simulink model "SF109A_ElecPwrCns"  (R2013b)
settings: Solver=FixedStepDiscrete  SolverMode=SingleTasking  StartTime=0.0  StopTime=1  FixedStep=0.002  RelTol=1e-3
values from neighbouring files (symbols this model uses):
  ARCHGLBPRM_HALFSQRT3_ULS_F32 = DataDict.Constant    [SF109A_ElecPwrCns_DataDict.m]
  ELECINPPWRESTIMHILIM_WATT_F32 = DataDict.Constant    [SF109A_ElecPwrCns_DataDict.m]
  ELECINPPWRESTIMLOLIM_WATT_F32 = DataDict.Constant    [SF109A_ElecPwrCns_DataDict.m]
  ElecPwrCnsCtrlrInpR = DataDict.Calibration    [SF109A_ElecPwrCns_DataDict.m]
  ElecPwrCnsPrstcPwrLoss = DataDict.Calibration    [SF109A_ElecPwrCns_DataDict.m]
  SPLYCURRESTIMHILIM_AMPR_F32 = DataDict.Constant    [SF109A_ElecPwrCns_DataDict.m]
  SPLYCURRESTIMLOLIM_AMPR_F32 = DataDict.Constant    [SF109A_ElecPwrCns_DataDict.m]
libraries: simulink x1
settings Model: LastModifiedBy=DZ1YRM
settings SolverCC: AutoInsertRateTranBlk=on  InsertRTBMode=Always
settings DataIOCC: LimitDataPoints=off  SaveFormat=Structure  ReturnWorkspaceOutputs=on
settings OptimizationCC: BlockReduction=off  InlineParams=on  ZeroExternalMemoryAtStartup=off  ZeroInternalMemoryAtStartup=off  OptimizeModelRefInitCode=on  LifeSpan=1
settings DebuggingCC: SignalInfNanChecking=error  SignalRangeChecking=warning  UnderspecifiedInitializationDetection=Simplified  SolverPrmCheckMsg=error  InheritedTsInSrcMsg=error  DiscreteInheritContinuousMsg=error  SingleTaskRateTransMsg=error  TasksWithSamePriorityMsg=error  SigSpecEnsureSampleTimeMsg=error  CheckMatrixSingularityMsg=error  ParameterUnderflowMsg=error  ParameterPrecisionLossMsg=error  ParameterTunabilityLossMsg=error  FixptConstUnderflowMsg=warning  FixptConstOverflowMsg=warning  VectorMatrixConversionMsg=error  SignalLabelMismatchMsg=error  UnconnectedInputMsg=error  UnconnectedOutputMsg=error  UnconnectedLineMsg=error  SFcnCompatibilityMsg=error  UniqueDataStoreMsg=warning  BusObjectLabelMismatch=error  RootOutportRequireBusObject=error  AssertControl=DisableAll  ModelReferenceIOMsg=error  ModelReferenceVersionMismatchMessage=warning  ModelReferenceIOMismatchMessage=error  ModelReferenceCSMismatchMessage=warning  ModelReferenceDataLoggingMessage=error  StateNameClashWarn=warning  StrictBusMsg=ErrorOnBusTreatedAsVector  NonBusSignalsTreatedAsBus=error  SFUnexpectedBacktrackingDiag=error  SFInvalidInputDataAccessInChartInitDiag=error  SFNoUnconditionalDefaultTransitionDiag=error  SFTransitionOutsideNaturalParentDiag=error  SFUnconditionalTransitionShadowingDiag=error  SFUndirectedBroadcastEventsDiag=error
settings ModelReferenceCC: ModelReferenceNumInstancesAllowed=Single
settings RTWCC: SystemTargetFile=autosar.tlc  GenCodeOnly=on  TemplateMakefile=ert_default_tmf  Description=AUTOSAR  GenerateReport=on  ProcessScript=autosar_make_rtw_hook  LaunchReport=on
settings CodeAppCC: GenerateComments=off  IgnoreCustomStorageClasses=off  CustomSymbolStrType=$N$R$M  CustomSymbolStrBlkIO=$N$M  SimulinkBlockComments=off
settings STFCustomTargetCC: ParMdlRefBuildCompliant=on  CompOptLevelCompliant=on  IncludeMdlTerminateFcn=off  CombineOutputUpdateFcns=on  SuppressErrorStatus=on  ERTFirstTimeCompliant=on  ERTCustomFileBanners=on  SupportNonFinite=off  SupportComplex=off  SupportContinuousTime=off  SupportNonInlinedSFcns=off  MATLABClassNameForMDSCustomization=Simulink.SoftwareTarget.ERTCustomization  AutosarCompliant=on  GRTInterface=off  SystemTargetFile=autosar.tlc
settings ERTTargetCC: CodeReplacementLibrary=ANSI_C  ConcurrentExecutionCompliant=off  IncludeMdlTerminateFcn=off  SuppressErrorStatus=on  SupportNonFinite=off  SupportComplex=off  ModelStepFunctionPrototypeControlCompliant=off  CPPClassGenCompliant=off  AutosarCompliant=on  InlinedParameterPlacement=NonHierarchical  ERTCustomFileTemplate=example_file_process.tlc  EnableUserReplacementTypes=on

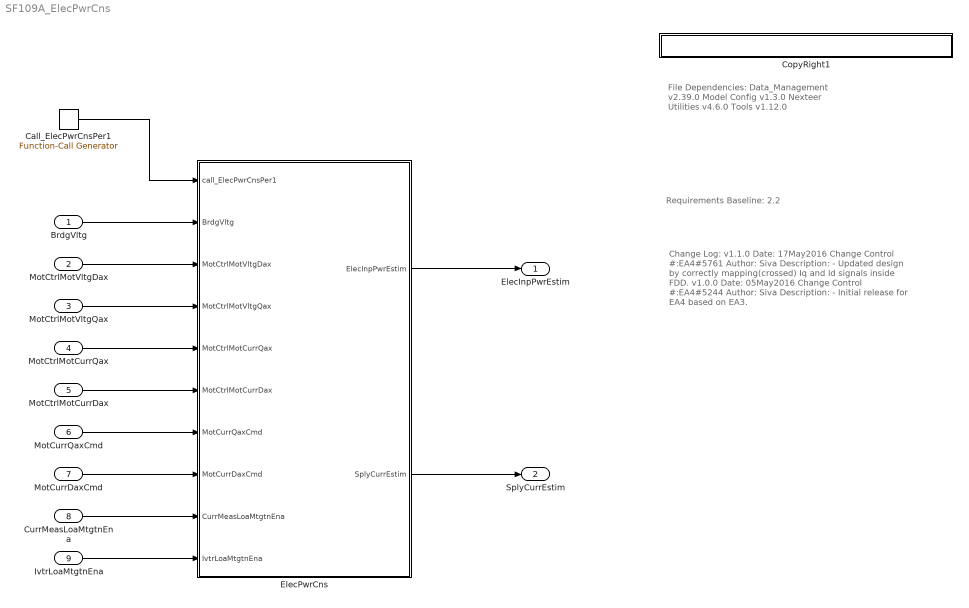
== system SF109A_ElecPwrCns ==
  note: File Dependencies:
      |
      | Data_Management v2.39.0
      | Model Config v1.3.0
      | Nexteer Utilities v4.6.0
      | Tools v1.12.0
  note: Requirements Baseline: 2.2
  note: Change Log:
      |
      | v1.1.0
      | Date: 17May2016
      | Change Control #:EA4#5761
      | Author: Siva
      | Description:
      | - Updated design by correctly mapping(crossed)
      |   Iq and Id signals inside FDD.
      |
      |
      | v1.0.0
      | Date: 05May2016
      | Change Control #:EA4#5244
      | Author: Siva
      | Description:
      | - Initial release for EA4 based on EA3.
  BrdgVltg : Inport
  MotCtrlMotVltgDax : Inport  Port=2
  MotCtrlMotVltgQax : Inport  Port=3
  MotCtrlMotCurrQax : Inport  Port=4
  MotCtrlMotCurrDax : Inport  Port=5
  MotCurrQaxCmd : Inport  Port=6
  MotCurrDaxCmd : Inport  Port=7
  CurrMeasLoaMtgtnEna : Inport  Port=8
  IvtrLoaMtgtnEna : Inport  Port=9
  Call_ElecPwrCnsPer1 : simulink/Ports & Subsystems/Function-Call Generator  sample_time=0.01  numberOfIterations=1
  CopyRight1 : Subsystem  Description=|  mask(Copyright Information){none=on}
      | Copyright info block.                                               
      |                                                                     
      | Place copyright information at the top of every subsystem in design.
      mask prompts: none "No parameters"
      mask help: Place copyright information at the top of every subsystem in design.
      mask Display:
      | NxtrConf = 'Nexteer Confidential';
      | 
      | sys = bdroot; %handle for the current model ("system")
      | first = get_param(sys,'Created');
      | if(isempty(first))
      |     first = datestr(now,'yyyy');
      | else
      |     first = first(end-3:end);  %year is last four digits
      | end
      | 
      | last = get_param(sys,'LastModifiedDate');
      | if isempty(last)
      |     last = datestr(now,'yyyy');
      | else
      |     last = last(end-3:end);
      | end
      | 
      | if strcmp(first,last)
      |     fprintf('%s -- Copyright %s Nexteer',NxtrConf,first)
      | else
      |     fprintf('%s -- %s%s- %s Nexteer',NxtrConf,char(169),first,last)
      | end
  ElecPwrCns : Subsystem
  ElecInpPwrEstim : Outport
  SplyCurrEstim : Outport  Port=2
  wires:
  ElecPwrCns/1(ElecInpPwrEstim) -> ElecInpPwrEstim/1
  ElecPwrCns/2(SplyCurrEstim) -> SplyCurrEstim/1
  Call_ElecPwrCnsPer1/1 -> ElecPwrCns/1(call_ElecPwrCnsPer1)
  MotCtrlMotVltgDax/1 -> ElecPwrCns/3(MotCtrlMotVltgDax)
  MotCtrlMotCurrDax/1 -> ElecPwrCns/6(MotCtrlMotCurrDax)
  CurrMeasLoaMtgtnEna/1 -> ElecPwrCns/9(CurrMeasLoaMtgtnEna)
  IvtrLoaMtgtnEna/1 -> ElecPwrCns/10(IvtrLoaMtgtnEna)
  MotCurrDaxCmd/1 -> ElecPwrCns/8(MotCurrDaxCmd)
  MotCtrlMotVltgQax/1 -> ElecPwrCns/4(MotCtrlMotVltgQax)
  MotCurrQaxCmd/1 -> ElecPwrCns/7(MotCurrQaxCmd)
  BrdgVltg/1 -> ElecPwrCns/2(BrdgVltg)
  MotCtrlMotCurrQax/1 -> ElecPwrCns/5(MotCtrlMotCurrQax)

== system SF109A_ElecPwrCns/CopyRight1 ==

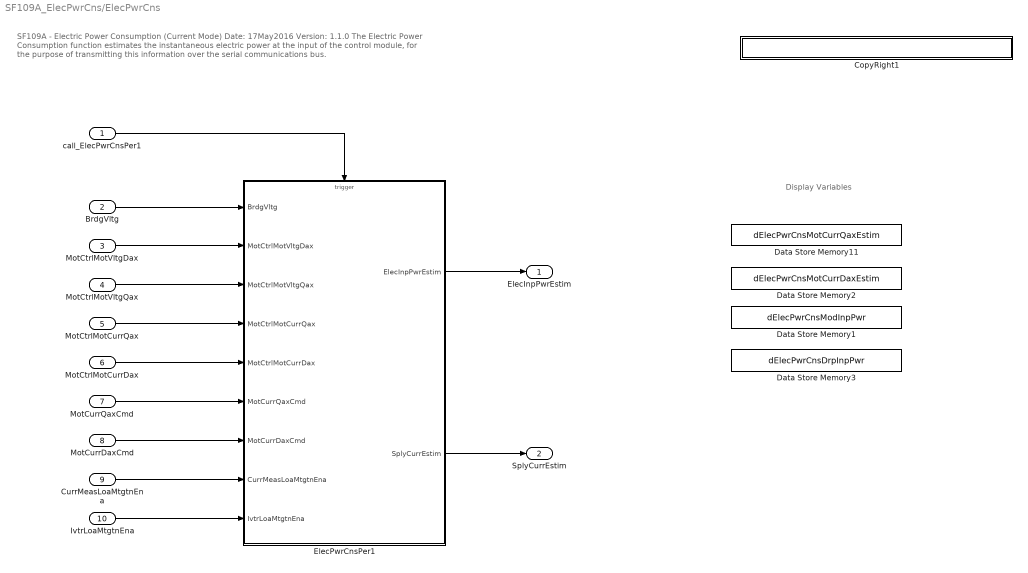
== system SF109A_ElecPwrCns/ElecPwrCns ==
  note: SF109A - Electric Power Consumption (Current Mode)
      | Date: 17May2016
      | Version: 1.1.0
      |
      | The Electric Power Consumption function estimates the instantaneous electric power at the input of the control module, for the purpose of transmitting this information
      | over the serial communications bus.
  note: Display Variables
  call_ElecPwrCnsPer1 : Inport  RequirementInfo={} %GIDa_da0c0603_8467_4dbe_980a_34e234362c51
  BrdgVltg : Inport  RequirementInfo="{'linktype_rmi_doors' '0000bb49 (/E-STEER Core/SubSystem Specifications/Application Functions/SF109A Electric Power Consumption )' '#SF109A_9' 'true' 'REQ:  SF109A_9' '' } %GIDa_cb384746_122a_4ac6_a5fd_4cc52726ee4f"  Port=2
  MotCtrlMotVltgDax : Inport  RequirementInfo="{'linktype_rmi_doors' '0000bb49 (/E-STEER Core/SubSystem Specifications/Application Functions/SF109A Electric Power Consumption )' '#SF109A_33' 'true' 'REQ:  SF109A_33' '' } %GIDa_0fee7270_14d1_452d_96a5_d6615c243f53"  Port=3
  MotCtrlMotVltgQax : Inport  RequirementInfo="{'linktype_rmi_doors' '0000bb49 (/E-STEER Core/SubSystem Specifications/Application Functions/SF109A Electric Power Consumption )' '#SF109A_32' 'true' 'REQ:  SF109A_32' '' } %GIDa_1366854d_cdb8_41c9_9ec7_b295409961f7"  Port=4
  MotCtrlMotCurrQax : Inport  RequirementInfo="{'linktype_rmi_doors' '0000bb49 (/E-STEER Core/SubSystem Specifications/Application Functions/SF109A Electric Power Consumption )' '#SF109A_34' 'true' 'REQ:  SF109A_34' '' } %GIDa_5e8aa2b9_a336_4638_be53_d49e57df33ab"  Port=5
  MotCtrlMotCurrDax : Inport  RequirementInfo="{'linktype_rmi_doors' '0000bb49 (/E-STEER Core/SubSystem Specifications/Application Functions/SF109A Electric Power Consumption )' '#SF109A_35' 'true' 'REQ:  SF109A_35' '' } %GIDa_7b415b12_f15f_4f64_9d4b_d3b77c1c51c9"  Port=6
  MotCurrQaxCmd : Inport  RequirementInfo="{'linktype_rmi_doors' '0000bb49 (/E-STEER Core/SubSystem Specifications/Application Functions/SF109A Electric Power Consumption )' '#SF109A_65' 'true' 'REQ:  SF109A_65' '' } %GIDa_17acaf13_cd99_4f03_882d_4ae5edd16e7f"  Port=7
  MotCurrDaxCmd : Inport  RequirementInfo="{'linktype_rmi_doors' '0000bb49 (/E-STEER Core/SubSystem Specifications/Application Functions/SF109A Electric Power Consumption )' '#SF109A_68' 'true' 'REQ:  SF109A_68' '' } %GIDa_e02e5d72_922e_4602_9ebf_785cee400470"  Port=8
  CurrMeasLoaMtgtnEna : Inport  RequirementInfo="{'linktype_rmi_doors' '0000bb49 (/E-STEER Core/SubSystem Specifications/Application Functions/SF109A Electric Power Consumption )' '#SF109A_67' 'true' 'REQ:  SF109A_67' '' } %GIDa_28f119ee_e929_47ec_805e_3810571495bd"  Port=9
  IvtrLoaMtgtnEna : Inport  RequirementInfo="{'linktype_rmi_doors' '0000bb49 (/E-STEER Core/SubSystem Specifications/Application Functions/SF109A Electric Power Consumption )' '#SF109A_66' 'true' 'REQ:  SF109A_66' '' } %GIDa_1221530d_3fe2_46fc_a8f2_438df6ced293"  Port=10
  CopyRight1 : Subsystem  Description=|  mask(Copyright Information){none=on}
      | Copyright info block.                                               
      |                                                                     
      | Place copyright information at the top of every subsystem in design.
      mask prompts: none "No parameters"
      mask help: Place copyright information at the top of every subsystem in design.
      mask Display:
      | NxtrConf = 'Nexteer Confidential';
      | 
      | sys = bdroot; %handle for the current model ("system")
      | first = get_param(sys,'Created');
      | if(isempty(first))
      |     first = datestr(now,'yyyy');
      | else
      |     first = first(end-3:end);  %year is last four digits
      | end
      | 
      | last = get_param(sys,'LastModifiedDate');
      | if isempty(last)
      |     last = datestr(now,'yyyy');
      | else
      |     last = last(end-3:end);
      | end
      | 
      | if strcmp(first,last)
      |     fprintf('%s -- Copyright %s Nexteer',NxtrConf,first)
      | else
      |     fprintf('%s -- %s%s- %s Nexteer',NxtrConf,char(169),first,last)
      | end
  Data Store Memory1 : DataStoreMemory  DataStoreName=dElecPwrCnsModInpPwr  StateMustResolveToSignalObject=on
  Data Store Memory11 : DataStoreMemory  DataStoreName=dElecPwrCnsMotCurrQaxEstim  StateMustResolveToSignalObject=on
  Data Store Memory2 : DataStoreMemory  DataStoreName=dElecPwrCnsMotCurrDaxEstim  StateMustResolveToSignalObject=on
  Data Store Memory3 : DataStoreMemory  DataStoreName=dElecPwrCnsDrpInpPwr  StateMustResolveToSignalObject=on
  ElecPwrCnsPer1 : Subsystem  RequirementInfo="{'linktype_rmi_doors' '0000bb49 (/E-STEER Core/SubSystem Specifications/Application Functions/SF109A Electric Power Consumption )' '#SF109A_58' 'true' 'REQ:  SF109A_58' '' ; 'linktype_rmi_doors' '0000bb49 (/E-STEER Core/SubSystem Specifications/Application Functions/SF109A Electric Power Consumption )' '#SF109A_73' 'true' 'REQ:  SF109A_73' '' ; 'linktype_rmi_doors' '0000bb49 (/E-STEER Core/SubSystem Specifications/Application Functions/SF109A Electric Power Consumption )' '#SF109A_72' 'true' 'REQ:  SF109A_72' '' } %GIDa_a5a46289_14d2_4e62_9199_b818a6881733"
  ElecInpPwrEstim : Outport  RequirementInfo="{'linktype_rmi_doors' '0000bb49 (/E-STEER Core/SubSystem Specifications/Application Functions/SF109A Electric Power Consumption )' '#SF109A_11' 'true' 'REQ:  SF109A_11' '' } %GIDa_77d0542b_de65_41ff_af8a_9807c86d67ac"
  SplyCurrEstim : Outport  RequirementInfo="{'linktype_rmi_doors' '0000bb49 (/E-STEER Core/SubSystem Specifications/Application Functions/SF109A Electric Power Consumption )' '#SF109A_36' 'true' 'REQ:  SF109A_36' '' } %GIDa_fef9d31a_76d5_40fc_b0ee_a68926f6c231"  Port=2
  wires:
  ElecPwrCnsPer1/1(ElecInpPwrEstim) -> ElecInpPwrEstim/1
  ElecPwrCnsPer1/2(SplyCurrEstim) -> SplyCurrEstim/1
  call_ElecPwrCnsPer1/1 -> ElecPwrCnsPer1/Trigger
  MotCtrlMotVltgDax/1 -> ElecPwrCnsPer1/2(MotCtrlMotVltgDax)
  BrdgVltg/1 -> ElecPwrCnsPer1/1(BrdgVltg)
  MotCurrQaxCmd/1 -> ElecPwrCnsPer1/6(MotCurrQaxCmd)
  MotCtrlMotVltgQax/1 -> ElecPwrCnsPer1/3(MotCtrlMotVltgQax)
  MotCtrlMotCurrQax/1 -> ElecPwrCnsPer1/4(MotCtrlMotCurrQax)
  IvtrLoaMtgtnEna/1 -> ElecPwrCnsPer1/9(IvtrLoaMtgtnEna)
  MotCtrlMotCurrDax/1 -> ElecPwrCnsPer1/5(MotCtrlMotCurrDax)
  MotCurrDaxCmd/1 -> ElecPwrCnsPer1/7(MotCurrDaxCmd)
  CurrMeasLoaMtgtnEna/1 -> ElecPwrCnsPer1/8(CurrMeasLoaMtgtnEna)

== system SF109A_ElecPwrCns/ElecPwrCns/CopyRight1 ==

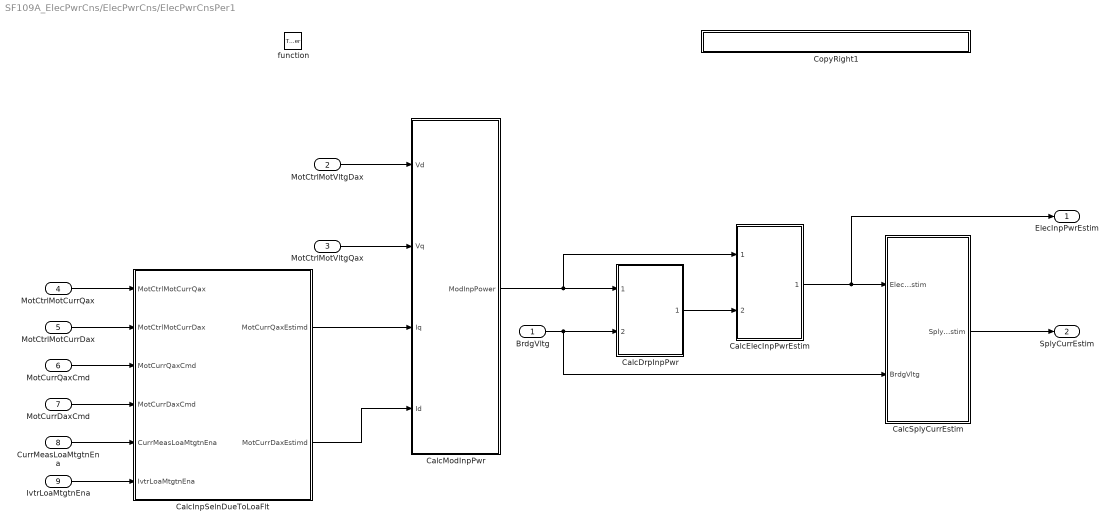
== system SF109A_ElecPwrCns/ElecPwrCns/ElecPwrCnsPer1 ==
  BrdgVltg : Inport
  MotCtrlMotVltgDax : Inport  Port=2
  MotCtrlMotVltgQax : Inport  Port=3
  MotCtrlMotCurrQax : Inport  Port=4
  MotCtrlMotCurrDax : Inport  Port=5
  MotCurrQaxCmd : Inport  Port=6
  MotCurrDaxCmd : Inport  Port=7
  CurrMeasLoaMtgtnEna : Inport  Port=8
  IvtrLoaMtgtnEna : Inport  Port=9
  function : TriggerPort  TriggerType=function-call
  CalcDrpInpPwr : Subsystem  RequirementInfo="{'linktype_rmi_doors' '0000bb49 (/E-STEER Core/SubSystem Specifications/Application Functions/SF109A Electric Power Consumption )' '#SF109A_44' 'true' 'REQ:  SF109A_44' '' } %GIDa_4f880266_c2b4_4393_8e8a_517d4de6c1f7"
  CalcElecInpPwrEstim : Subsystem  RequirementInfo="{'linktype_rmi_doors' '0000bb49 (/E-STEER Core/SubSystem Specifications/Application Functions/SF109A Electric Power Consumption )' '#SF109A_49' 'true' 'REQ:  SF109A_49' '' } %GIDa_d54b4fcf_36ba_4a63_99c8_8362976887f3"
  CalcInpSelnDueToLoaFlt : Subsystem  RequirementInfo="{'linktype_rmi_doors' '0000bb49 (/E-STEER Core/SubSystem Specifications/Application Functions/SF109A Electric Power Consumption )' '#SF109A_59' 'true' 'REQ:  SF109A_59' '' } %GIDa_3a34917a_fcc8_409d_aaef_3e9b257a480a"
  CalcModInpPwr : Subsystem  RequirementInfo="{'linktype_rmi_doors' '0000bb49 (/E-STEER Core/SubSystem Specifications/Application Functions/SF109A Electric Power Consumption )' '#SF109A_60' 'true' 'REQ:  SF109A_60' '' } %GIDa_35639a43_10bc_4a66_aa79_a3e46d540002"
  CalcSplyCurrEstim : Subsystem  RequirementInfo="{'linktype_rmi_doors' '0000bb49 (/E-STEER Core/SubSystem Specifications/Application Functions/SF109A Electric Power Consumption )' '#SF109A_70' 'true' 'REQ:  SF109A_70' '' } %GIDa_e9e41846_670c_407c_9959_3b9f2f44b6c5"
  CopyRight1 : Subsystem  Description=|  mask(Copyright Information){none=on}
      | Copyright info block.                                               
      |                                                                     
      | Place copyright information at the top of every subsystem in design.
      mask prompts: none "No parameters"
      mask help: Place copyright information at the top of every subsystem in design.
      mask Display:
      | NxtrConf = 'Nexteer Confidential';
      | 
      | sys = bdroot; %handle for the current model ("system")
      | first = get_param(sys,'Created');
      | if(isempty(first))
      |     first = datestr(now,'yyyy');
      | else
      |     first = first(end-3:end);  %year is last four digits
      | end
      | 
      | last = get_param(sys,'LastModifiedDate');
      | if isempty(last)
      |     last = datestr(now,'yyyy');
      | else
      |     last = last(end-3:end);
      | end
      | 
      | if strcmp(first,last)
      |     fprintf('%s -- Copyright %s Nexteer',NxtrConf,first)
      | else
      |     fprintf('%s -- %s%s- %s Nexteer',NxtrConf,char(169),first,last)
      | end
  ElecInpPwrEstim : Outport
  SplyCurrEstim : Outport  Port=2
  wires:
  CalcModInpPwr/1(ModInpPower) -> CalcDrpInpPwr/1(ModInpPwr), CalcElecInpPwrEstim/1(ModInpPwr)
  MotCtrlMotVltgDax/1 -> CalcModInpPwr/1(Vd)
  MotCtrlMotVltgQax/1 -> CalcModInpPwr/2(Vq)
  BrdgVltg/1 -> CalcSplyCurrEstim/2(BrdgVltg), CalcDrpInpPwr/2(BrdgVltg)
  MotCtrlMotCurrDax/1 -> CalcInpSelnDueToLoaFlt/2(MotCtrlMotCurrDax)
  MotCurrDaxCmd/1 -> CalcInpSelnDueToLoaFlt/4(MotCurrDaxCmd)
  MotCtrlMotCurrQax/1 -> CalcInpSelnDueToLoaFlt/1(MotCtrlMotCurrQax)
  MotCurrQaxCmd/1 -> CalcInpSelnDueToLoaFlt/3(MotCurrQaxCmd)
  CalcSplyCurrEstim/1(SplyCurrEstim) -> SplyCurrEstim/1
  CurrMeasLoaMtgtnEna/1 -> CalcInpSelnDueToLoaFlt/5(CurrMeasLoaMtgtnEna)
  IvtrLoaMtgtnEna/1 -> CalcInpSelnDueToLoaFlt/6(IvtrLoaMtgtnEna)
  CalcElecInpPwrEstim/1(ElecInpPwrEstim) -> ElecInpPwrEstim/1, CalcSplyCurrEstim/1(ElecInpPwrEstim)
  CalcDrpInpPwr/1(DrpInpPwr) -> CalcElecInpPwrEstim/2(DropInpPwr)
  CalcInpSelnDueToLoaFlt/1(MotCurrQaxEstimd) -> CalcModInpPwr/3(Iq)
  CalcInpSelnDueToLoaFlt/2(MotCurrDaxEstimd) -> CalcModInpPwr/4(Id)

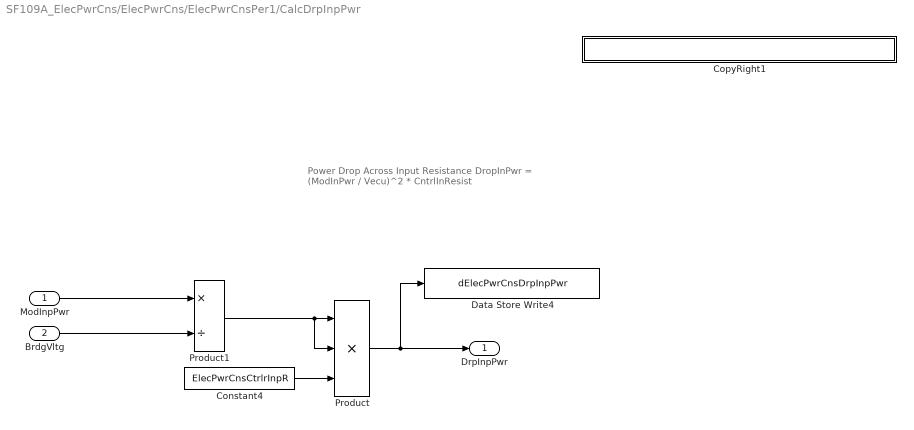
== system SF109A_ElecPwrCns/ElecPwrCns/ElecPwrCnsPer1/CalcDrpInpPwr ==
  note: Power Drop Across Input Resistance
      |
      | DropInPwr = (ModInPwr / Vecu)^2 * CntrlInResist
  ModInpPwr : Inport
  BrdgVltg : Inport  Port=2
  Constant4 : Constant  RequirementInfo="{'linktype_rmi_doors' '0000bb49 (/E-STEER Core/SubSystem Specifications/Application Functions/SF109A Electric Power Consumption )' '#SF109A_61' 'true' 'REQ:  SF109A_61' '' } %GIDa_ccdd9ab8_df5d_4409_97d9_316a4dc3a4df"  Value=ElecPwrCnsCtrlrInpR
  CopyRight1 : Subsystem  Description=|  mask(Copyright Information){none=on}
      | Copyright info block.                                               
      |                                                                     
      | Place copyright information at the top of every subsystem in design.
      mask prompts: none "No parameters"
      mask help: Place copyright information at the top of every subsystem in design.
      mask Display:
      | NxtrConf = 'Nexteer Confidential';
      | 
      | sys = bdroot; %handle for the current model ("system")
      | first = get_param(sys,'Created');
      | if(isempty(first))
      |     first = datestr(now,'yyyy');
      | else
      |     first = first(end-3:end);  %year is last four digits
      | end
      | 
      | last = get_param(sys,'LastModifiedDate');
      | if isempty(last)
      |     last = datestr(now,'yyyy');
      | else
      |     last = last(end-3:end);
      | end
      | 
      | if strcmp(first,last)
      |     fprintf('%s -- Copyright %s Nexteer',NxtrConf,first)
      | else
      |     fprintf('%s -- %s%s- %s Nexteer',NxtrConf,char(169),first,last)
      | end
  Data Store Write4 : DataStoreWrite  DataStoreName=dElecPwrCnsDrpInpPwr
  Product : Product  RequirementInfo="{'linktype_rmi_doors' '0000bb49 (/E-STEER Core/SubSystem Specifications/Application Functions/SF109A Electric Power Consumption )' '#SF109A_44' 'true' 'REQ:  SF109A_44' '' } %GIDa_4d888400_6a5b_416d_8968_0d46b2df3211"  Inputs=3  RndMeth=Zero
  Product1 : Product  RequirementInfo="{'linktype_rmi_doors' '0000bb49 (/E-STEER Core/SubSystem Specifications/Application Functions/SF109A Electric Power Consumption )' '#SF109A_44' 'true' 'REQ:  SF109A_44' '' } %GIDa_ac85e963_71f0_4a43_ae6a_18c02b609f26"  Inputs=*/  RndMeth=Zero
  DrpInpPwr : Outport  RequirementInfo={} %GIDa_90e28425_22d1_477b_80e2_71849123ef87
  wires:
  Product/1 -> Data Store Write4/1, DrpInpPwr/1
  Product1/1 -> Product/2, Product/1
  BrdgVltg/1 -> Product1/2
  ModInpPwr/1 -> Product1/1
  Constant4/1 -> Product/3

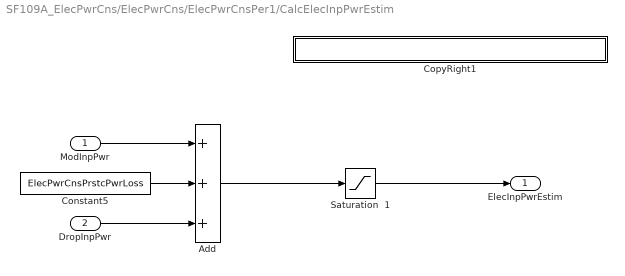
== system SF109A_ElecPwrCns/ElecPwrCns/ElecPwrCnsPer1/CalcElecInpPwrEstim ==
  ModInpPwr : Inport
  DropInpPwr : Inport  Port=2
  Add : Sum  RequirementInfo="{'linktype_rmi_doors' '0000bb49 (/E-STEER Core/SubSystem Specifications/Application Functions/SF109A Electric Power Consumption )' '#SF109A_49' 'true' 'REQ:  SF109A_49' '' } %GIDa_f386c1dc_c79d_4dbf_a4c8_3a168f40c696"  Inputs=3
  Constant5 : Constant  RequirementInfo="{'linktype_rmi_doors' '0000bb49 (/E-STEER Core/SubSystem Specifications/Application Functions/SF109A Electric Power Consumption )' '#SF109A_49' 'true' 'REQ:  SF109A_49' '' ; 'linktype_rmi_doors' '0000bb49 (/E-STEER Core/SubSystem Specifications/Application Functions/SF109A Electric Power Consumption )' '#SF109A_62' 'true' 'REQ:  SF109A_62' '' } %GIDa_3af8c988_3fde_466a_8f42_d9fcd1893325"  Value=ElecPwrCnsPrstcPwrLoss
  CopyRight1 : Subsystem  Description=|  mask(Copyright Information){none=on}
      | Copyright info block.                                               
      |                                                                     
      | Place copyright information at the top of every subsystem in design.
      mask prompts: none "No parameters"
      mask help: Place copyright information at the top of every subsystem in design.
      mask Display:
      | NxtrConf = 'Nexteer Confidential';
      | 
      | sys = bdroot; %handle for the current model ("system")
      | first = get_param(sys,'Created');
      | if(isempty(first))
      |     first = datestr(now,'yyyy');
      | else
      |     first = first(end-3:end);  %year is last four digits
      | end
      | 
      | last = get_param(sys,'LastModifiedDate');
      | if isempty(last)
      |     last = datestr(now,'yyyy');
      | else
      |     last = last(end-3:end);
      | end
      | 
      | if strcmp(first,last)
      |     fprintf('%s -- Copyright %s Nexteer',NxtrConf,first)
      | else
      |     fprintf('%s -- %s%s- %s Nexteer',NxtrConf,char(169),first,last)
      | end
  Saturation  1 : Saturate  RequirementInfo="{'linktype_rmi_doors' '0000bb49 (/E-STEER Core/SubSystem Specifications/Application Functions/SF109A Electric Power Consumption )' '#SF109A_63' 'true' 'REQ:  SF109A_63' '' } %GIDa_0e9dd2a2_e5f0_4a7d_bff6_e5ae1bc1844d"  UpperLimit=ELECINPPWRESTIMHILIM_WATT_F32  LowerLimit=ELECINPPWRESTIMLOLIM_WATT_F32
      settings: AttributesFormatString=|
      | Lower Limit: %<LowerLimit>
      | Upper Limit: %<UpperLimit>
  ElecInpPwrEstim : Outport
  wires:
  Add/1 -> Saturation  1/1
  DropInpPwr/1 -> Add/3
  Constant5/1 -> Add/2
  ModInpPwr/1 -> Add/1
  Saturation  1/1 -> ElecInpPwrEstim/1

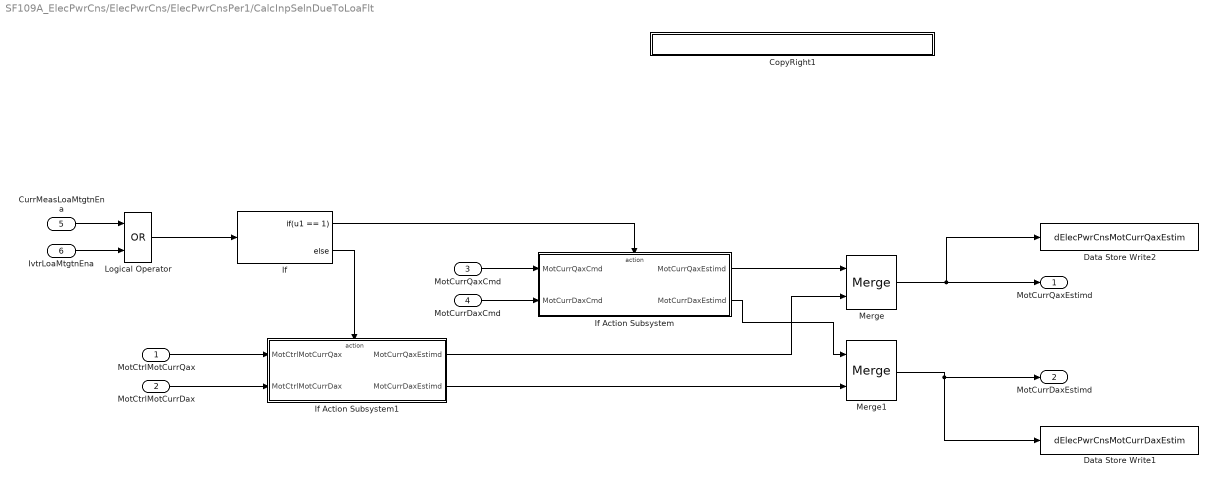
== system SF109A_ElecPwrCns/ElecPwrCns/ElecPwrCnsPer1/CalcInpSelnDueToLoaFlt ==
  MotCtrlMotCurrQax : Inport
  MotCtrlMotCurrDax : Inport  Port=2
  MotCurrQaxCmd : Inport  RequirementInfo={} %GIDa_84596482_d14b_44bc_bcfc_52e1b1c4b436  Port=3
  MotCurrDaxCmd : Inport  RequirementInfo={} %GIDa_c4f65746_217c_4e3d_8a9e_d4b25fed7d57  Port=4
  CurrMeasLoaMtgtnEna : Inport  Port=5
  IvtrLoaMtgtnEna : Inport  Port=6
  CopyRight1 : Subsystem  Description=|  mask(Copyright Information){none=on}
      | Copyright info block.                                               
      |                                                                     
      | Place copyright information at the top of every subsystem in design.
      mask prompts: none "No parameters"
      mask help: Place copyright information at the top of every subsystem in design.
      mask Display:
      | NxtrConf = 'Nexteer Confidential';
      | 
      | sys = bdroot; %handle for the current model ("system")
      | first = get_param(sys,'Created');
      | if(isempty(first))
      |     first = datestr(now,'yyyy');
      | else
      |     first = first(end-3:end);  %year is last four digits
      | end
      | 
      | last = get_param(sys,'LastModifiedDate');
      | if isempty(last)
      |     last = datestr(now,'yyyy');
      | else
      |     last = last(end-3:end);
      | end
      | 
      | if strcmp(first,last)
      |     fprintf('%s -- Copyright %s Nexteer',NxtrConf,first)
      | else
      |     fprintf('%s -- %s%s- %s Nexteer',NxtrConf,char(169),first,last)
      | end
  Data Store Write1 : DataStoreWrite  DataStoreName=dElecPwrCnsMotCurrDaxEstim
  Data Store Write2 : DataStoreWrite  DataStoreName=dElecPwrCnsMotCurrQaxEstim
  If : If  RequirementInfo="{'linktype_rmi_doors' '0000bb49 (/E-STEER Core/SubSystem Specifications/Application Functions/SF109A Electric Power Consumption )' '#SF109A_59' 'true' 'REQ:  SF109A_59' '' } %GIDa_4daf5aca_daee_4c41_8365_78956bb4ead0"  IfExpression=u1 == 1
  If Action Subsystem : Subsystem  RequirementInfo="{'linktype_rmi_doors' '0000bb49 (/E-STEER Core/SubSystem Specifications/Application Functions/SF109A Electric Power Consumption )' '#SF109A_59' 'true' 'REQ:  SF109A_59' '' } %GIDa_6f703d4f_f0b0_4b81_a2bb_13839db3fe0c"  TreatAsAtomicUnit=on
  If Action Subsystem1 : Subsystem  RequirementInfo="{'linktype_rmi_doors' '0000bb49 (/E-STEER Core/SubSystem Specifications/Application Functions/SF109A Electric Power Consumption )' '#SF109A_59' 'true' 'REQ:  SF109A_59' '' } %GIDa_92e9d284_51b6_4370_bf51_7ea5acba6145"  TreatAsAtomicUnit=on
  Logical Operator : Logic  RequirementInfo="{'linktype_rmi_doors' '0000bb49 (/E-STEER Core/SubSystem Specifications/Application Functions/SF109A Electric Power Consumption )' '#SF109A_59' 'true' 'REQ:  SF109A_59' '' } %GIDa_7cbabdd9_e684_4d82_a01a_66a26bc33d8d"  Operator=OR  AllPortsSameDT=off  OutDataTypeStr=boolean
  Merge : Merge  RequirementInfo={} %GIDa_f7d16e22_aae1_4531_ab34_e0e60118ee2f
  Merge1 : Merge  RequirementInfo={} %GIDa_97831f1b_d76e_4766_b838_72f628fd3eac
  MotCurrQaxEstimd : Outport
  MotCurrDaxEstimd : Outport  Port=2
  wires:
  Merge/1 -> Data Store Write2/1, MotCurrQaxEstimd/1
  If/1 -> If Action Subsystem/Action
  If/2 -> If Action Subsystem1/Action
  MotCurrQaxCmd/1 -> If Action Subsystem/1(MotCurrQaxCmd)
  If Action Subsystem/1(MotCurrQaxEstimd) -> Merge/1
  If Action Subsystem1/1(MotCurrQaxEstimd) -> Merge/2
  MotCtrlMotCurrQax/1 -> If Action Subsystem1/1(MotCtrlMotCurrQax)
  CurrMeasLoaMtgtnEna/1 -> Logical Operator/1
  IvtrLoaMtgtnEna/1 -> Logical Operator/2
  Logical Operator/1 -> If/1
  MotCurrDaxCmd/1 -> If Action Subsystem/2(MotCurrDaxCmd)
  MotCtrlMotCurrDax/1 -> If Action Subsystem1/2(MotCtrlMotCurrDax)
  If Action Subsystem/2(MotCurrDaxEstimd) -> Merge1/1
  If Action Subsystem1/2(MotCurrDaxEstimd) -> Merge1/2
  Merge1/1 -> Data Store Write1/1, MotCurrDaxEstimd/1

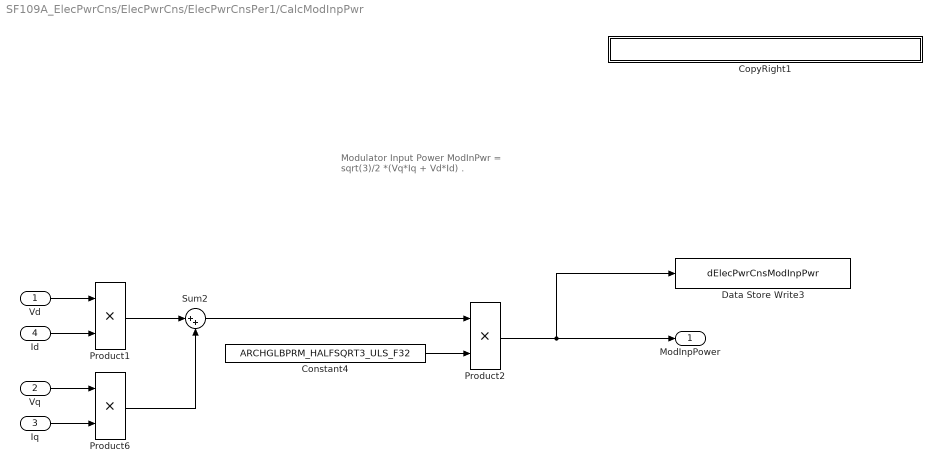
== system SF109A_ElecPwrCns/ElecPwrCns/ElecPwrCnsPer1/CalcModInpPwr ==
  note: Modulator Input Power
      |
      | ModInPwr = sqrt(3)/2 *(Vq*Iq + Vd*Id)
      | .
  Vd : Inport
  Vq : Inport  Port=2
  Iq : Inport  Port=3
  Id : Inport  Port=4
  Constant4 : Constant  RequirementInfo="{'linktype_rmi_doors' '0000bb49 (/E-STEER Core/SubSystem Specifications/Application Functions/SF109A Electric Power Consumption )' '#SF109A_60' 'true' 'REQ:  SF109A_60' '' } %GIDa_2f0e32e0_f631_467e_b8de_32a9adf53d14"  Value=ARCHGLBPRM_HALFSQRT3_ULS_F32
  CopyRight1 : Subsystem  Description=|  mask(Copyright Information){none=on}
      | Copyright info block.                                               
      |                                                                     
      | Place copyright information at the top of every subsystem in design.
      mask prompts: none "No parameters"
      mask help: Place copyright information at the top of every subsystem in design.
      mask Display:
      | NxtrConf = 'Nexteer Confidential';
      | 
      | sys = bdroot; %handle for the current model ("system")
      | first = get_param(sys,'Created');
      | if(isempty(first))
      |     first = datestr(now,'yyyy');
      | else
      |     first = first(end-3:end);  %year is last four digits
      | end
      | 
      | last = get_param(sys,'LastModifiedDate');
      | if isempty(last)
      |     last = datestr(now,'yyyy');
      | else
      |     last = last(end-3:end);
      | end
      | 
      | if strcmp(first,last)
      |     fprintf('%s -- Copyright %s Nexteer',NxtrConf,first)
      | else
      |     fprintf('%s -- %s%s- %s Nexteer',NxtrConf,char(169),first,last)
      | end
  Data Store Write3 : DataStoreWrite  DataStoreName=dElecPwrCnsModInpPwr
  Product1 : Product  RequirementInfo="{'linktype_rmi_doors' '0000bb49 (/E-STEER Core/SubSystem Specifications/Application Functions/SF109A Electric Power Consumption )' '#SF109A_60' 'true' 'REQ:  SF109A_60' '' } %GIDa_842b6729_5424_4ba7_a45e_36e0f9165d11"  RndMeth=Zero
  Product2 : Product  RequirementInfo="{'linktype_rmi_doors' '0000bb49 (/E-STEER Core/SubSystem Specifications/Application Functions/SF109A Electric Power Consumption )' '#SF109A_60' 'true' 'REQ:  SF109A_60' '' } %GIDa_d3535dab_61fe_4be6_9356_27768f395b77"  RndMeth=Zero
  Product6 : Product  RequirementInfo="{'linktype_rmi_doors' '0000bb49 (/E-STEER Core/SubSystem Specifications/Application Functions/SF109A Electric Power Consumption )' '#SF109A_60' 'true' 'REQ:  SF109A_60' '' } %GIDa_b0fc09be_30dd_48ca_884f_0e907df93816"  RndMeth=Zero
  Sum2 : Sum  RequirementInfo="{'linktype_rmi_doors' '0000bb49 (/E-STEER Core/SubSystem Specifications/Application Functions/SF109A Electric Power Consumption )' '#SF109A_60' 'true' 'REQ:  SF109A_60' '' } %GIDa_486ee27e_b56a_4899_b6bf_458eba889f7d"  Inputs=|++
  ModInpPower : Outport
  wires:
  Product2/1 -> Data Store Write3/1, ModInpPower/1
  Product1/1 -> Sum2/1
  Product6/1 -> Sum2/2
  Sum2/1 -> Product2/1
  Vd/1 -> Product1/1
  Id/1 -> Product1/2
  Vq/1 -> Product6/1
  Iq/1 -> Product6/2
  Constant4/1 -> Product2/2

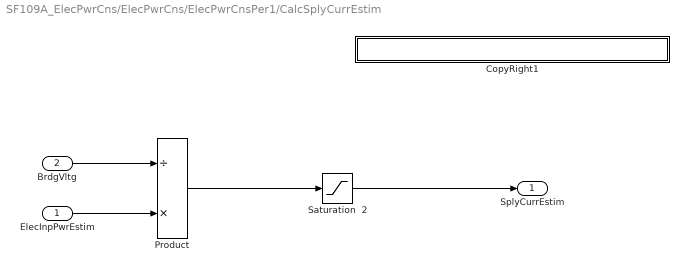
== system SF109A_ElecPwrCns/ElecPwrCns/ElecPwrCnsPer1/CalcSplyCurrEstim ==
  ElecInpPwrEstim : Inport
  BrdgVltg : Inport  Port=2
  CopyRight1 : Subsystem  Description=|  mask(Copyright Information){none=on}
      | Copyright info block.                                               
      |                                                                     
      | Place copyright information at the top of every subsystem in design.
      mask prompts: none "No parameters"
      mask help: Place copyright information at the top of every subsystem in design.
      mask Display:
      | NxtrConf = 'Nexteer Confidential';
      | 
      | sys = bdroot; %handle for the current model ("system")
      | first = get_param(sys,'Created');
      | if(isempty(first))
      |     first = datestr(now,'yyyy');
      | else
      |     first = first(end-3:end);  %year is last four digits
      | end
      | 
      | last = get_param(sys,'LastModifiedDate');
      | if isempty(last)
      |     last = datestr(now,'yyyy');
      | else
      |     last = last(end-3:end);
      | end
      | 
      | if strcmp(first,last)
      |     fprintf('%s -- Copyright %s Nexteer',NxtrConf,first)
      | else
      |     fprintf('%s -- %s%s- %s Nexteer',NxtrConf,char(169),first,last)
      | end
  Product : Product  RequirementInfo="{'linktype_rmi_doors' '0000bb49 (/E-STEER Core/SubSystem Specifications/Application Functions/SF109A Electric Power Consumption )' '#SF109A_70' 'true' 'REQ:  SF109A_70' '' } %GIDa_24a4bfdd_0f07_4e2c_9228_c53345fab438"  Inputs=/*  RndMeth=Zero
  Saturation  2 : Saturate  RequirementInfo="{'linktype_rmi_doors' '0000bb49 (/E-STEER Core/SubSystem Specifications/Application Functions/SF109A Electric Power Consumption )' '#SF109A_69' 'true' 'REQ:  SF109A_69' '' } %GIDa_969f665f_a3c9_4ff2_867a_965ec286eea1"  UpperLimit=SPLYCURRESTIMHILIM_AMPR_F32  LowerLimit=SPLYCURRESTIMLOLIM_AMPR_F32
      settings: AttributesFormatString=|
      | Lower Limit: %<LowerLimit>
      | Upper Limit: %<UpperLimit>
  SplyCurrEstim : Outport
  wires:
  Product/1 -> Saturation  2/1
  ElecInpPwrEstim/1 -> Product/2
  BrdgVltg/1 -> Product/1
  Saturation  2/1 -> SplyCurrEstim/1

== system SF109A_ElecPwrCns/ElecPwrCns/ElecPwrCnsPer1/CopyRight1 ==

== system SF109A_ElecPwrCns/ElecPwrCns/ElecPwrCnsPer1/CalcDrpInpPwr/CopyRight1 ==

== system SF109A_ElecPwrCns/ElecPwrCns/ElecPwrCnsPer1/CalcElecInpPwrEstim/CopyRight1 ==

== system SF109A_ElecPwrCns/ElecPwrCns/ElecPwrCnsPer1/CalcInpSelnDueToLoaFlt/CopyRight1 ==

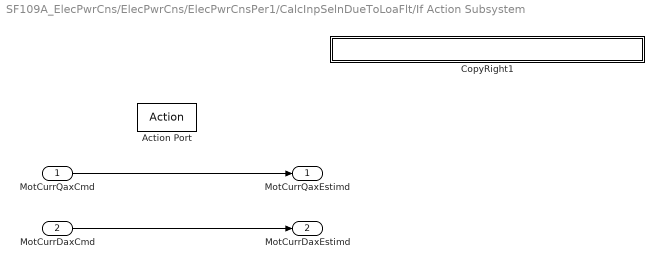
== system SF109A_ElecPwrCns/ElecPwrCns/ElecPwrCnsPer1/CalcInpSelnDueToLoaFlt/If Action Subsystem ==
  MotCurrQaxCmd : Inport
  MotCurrDaxCmd : Inport  Port=2
  Action Port : ActionPort  ActionType=then
  CopyRight1 : Subsystem  Description=|  mask(Copyright Information){none=on}
      | Copyright info block.                                               
      |                                                                     
      | Place copyright information at the top of every subsystem in design.
      mask prompts: none "No parameters"
      mask help: Place copyright information at the top of every subsystem in design.
      mask Display:
      | NxtrConf = 'Nexteer Confidential';
      | 
      | sys = bdroot; %handle for the current model ("system")
      | first = get_param(sys,'Created');
      | if(isempty(first))
      |     first = datestr(now,'yyyy');
      | else
      |     first = first(end-3:end);  %year is last four digits
      | end
      | 
      | last = get_param(sys,'LastModifiedDate');
      | if isempty(last)
      |     last = datestr(now,'yyyy');
      | else
      |     last = last(end-3:end);
      | end
      | 
      | if strcmp(first,last)
      |     fprintf('%s -- Copyright %s Nexteer',NxtrConf,first)
      | else
      |     fprintf('%s -- %s%s- %s Nexteer',NxtrConf,char(169),first,last)
      | end
  MotCurrQaxEstimd : Outport
  MotCurrDaxEstimd : Outport  Port=2
  wires:
  MotCurrQaxCmd/1 -> MotCurrQaxEstimd/1
  MotCurrDaxCmd/1 -> MotCurrDaxEstimd/1

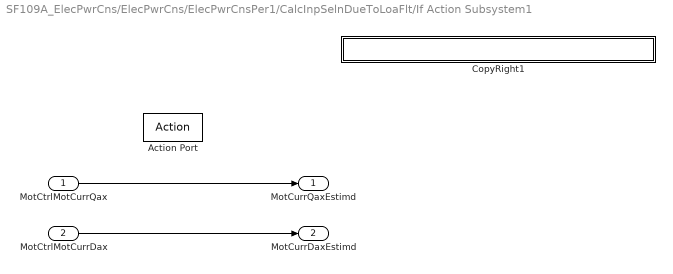
== system SF109A_ElecPwrCns/ElecPwrCns/ElecPwrCnsPer1/CalcInpSelnDueToLoaFlt/If Action Subsystem1 ==
  MotCtrlMotCurrQax : Inport
  MotCtrlMotCurrDax : Inport  Port=2
  Action Port : ActionPort  ActionType=else
  CopyRight1 : Subsystem  Description=|  mask(Copyright Information){none=on}
      | Copyright info block.                                               
      |                                                                     
      | Place copyright information at the top of every subsystem in design.
      mask prompts: none "No parameters"
      mask help: Place copyright information at the top of every subsystem in design.
      mask Display:
      | NxtrConf = 'Nexteer Confidential';
      | 
      | sys = bdroot; %handle for the current model ("system")
      | first = get_param(sys,'Created');
      | if(isempty(first))
      |     first = datestr(now,'yyyy');
      | else
      |     first = first(end-3:end);  %year is last four digits
      | end
      | 
      | last = get_param(sys,'LastModifiedDate');
      | if isempty(last)
      |     last = datestr(now,'yyyy');
      | else
      |     last = last(end-3:end);
      | end
      | 
      | if strcmp(first,last)
      |     fprintf('%s -- Copyright %s Nexteer',NxtrConf,first)
      | else
      |     fprintf('%s -- %s%s- %s Nexteer',NxtrConf,char(169),first,last)
      | end
  MotCurrQaxEstimd : Outport
  MotCurrDaxEstimd : Outport  Port=2
  wires:
  MotCtrlMotCurrQax/1 -> MotCurrQaxEstimd/1
  MotCtrlMotCurrDax/1 -> MotCurrDaxEstimd/1

== system SF109A_ElecPwrCns/ElecPwrCns/ElecPwrCnsPer1/CalcModInpPwr/CopyRight1 ==

== system SF109A_ElecPwrCns/ElecPwrCns/ElecPwrCnsPer1/CalcSplyCurrEstim/CopyRight1 ==

== system SF109A_ElecPwrCns/ElecPwrCns/ElecPwrCnsPer1/CalcInpSelnDueToLoaFlt/If Action Subsystem/CopyRight1 ==

== system SF109A_ElecPwrCns/ElecPwrCns/ElecPwrCnsPer1/CalcInpSelnDueToLoaFlt/If Action Subsystem1/CopyRight1 ==
